simulink model "bang"  (Simulink 7.0)
settings: Solver=ode45  StartTime=0.0  StopTime=abs(xdot/N)  RelTol=1e-6
values from neighbouring files (symbols this model uses):
  N = 1.00    (= 1)    [f_tos.m]
undefined symbols (not defined in the file or in its folder): x, xdot
settings Model: Creator=abbas  LastModifiedBy=abbas
settings OptimizationCC: InlineInvariantSignals=on
settings DebuggingCC: SaveWithParameterizedLinksMsg=none  SignalResolutionControl=TryResolveAllWithWarning  SolverPrmCheckMsg=none  MultiTaskDSMMsg=warning  MultiTaskCondExecSysMsg=none  StrictBusMsg=None
settings RTWCC: IncludeERTFirstTime=on
settings GRTTargetCC: TargetFcnLib=ansi_tfl_tmw.mat

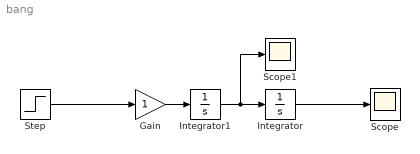
== system bang ==
  Gain : Gain  ParameterDataType=sfix(16)  ParameterScaling=2^0  OutDataType=sfix(16)  OutScaling=2^0
  Integrator : Integrator  InitialCondition=x
  Integrator1 : Integrator  InitialCondition=xdot
  Scope : Scope
      settings: SaveName=xbang  DataFormat=Array
  Scope1 : Scope
      settings: SaveName=xdotbang  DataFormat=Array
  Step : Step  Time=0  After=N  SampleTime=0
  wires:
  Integrator1/1 -> Integrator/1, Scope1/1
  Integrator/1 -> Scope/1
  Gain/1 -> Integrator1/1
  Step/1 -> Gain/1
